simulink model "Lab5_1"  (R2023a)
settings: Solver=FixedStepDiscrete  StartTime=0.0  StopTime=A.len*16 + 52  FixedStep=1  RelTol=1e-3
PostLoadFcn:
  | A = DEScfg_axi('$0102040810204080', 'This is a default input - make it your own!', 'encrypt')
undefined symbols (not defined in the file): AXI4, Lite, xc7z020clg484
libraries: hdlBasic x260, vmcUtilities x1
(part 1 of 2)
settings Model: Creator=gunnarg  LastModifiedBy=robg
settings SolverCC: AlgebraicLoopSolver=TrustRegion
settings DataIOCC: LimitDataPoints=on  SaveFormat=Array  ReturnWorkspaceOutputs=off
settings OptimizationCC: LifeSpan=inf
settings DebuggingCC: SolverPrmCheckMsg=warning  UnconnectedInputMsg=warning  UnconnectedOutputMsg=warning  UnconnectedLineMsg=warning  SFUnexpectedBacktrackingDiag=warning  SFNoUnconditionalDefaultTransitionDiag=warning  ArithmeticOperatorsInVariantConditions=warning
settings HardwareCC: ProdBitPerPointer=32  ProdBitPerSizeT=32  ProdBitPerPtrDiffT=32  ProdLargestAtomicFloat=None  ProdIntDivRoundTo=Undefined  ProdEndianess=Unspecified  ProdWordSize=32  ProdHWDeviceType=32-bit Generic
settings ModelReferenceCC: EnableRefExpFcnMdlSchedulingChecks=on  PropagateSignalLabelsOutOfModel=off
settings SFSimCC: SimUseLocalCustomCode=off  CustomCodeUndefinedFunction=UseInterfaceOnly
settings RTWCC: RTWUseLocalCustomCode=off  DLArmComputeVersion=19.05
settings CodeAppCC: StateflowObjectComments=on
settings GRTTargetCC: TargetLangStandard=C89/C90 (ANSI)
settings ConfigComp: CovMetricSettings=dw  CovSaveCumulativeToWorkspaceVar=on  CovSaveSingleToWorkspaceVar=on  CovExternalEMLEnable=off  CovSFcnEnable=off

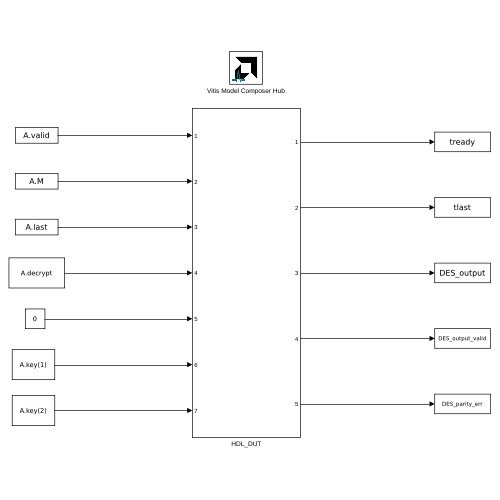
[thumbnail: Simulink's stored preview of the top-level diagram]
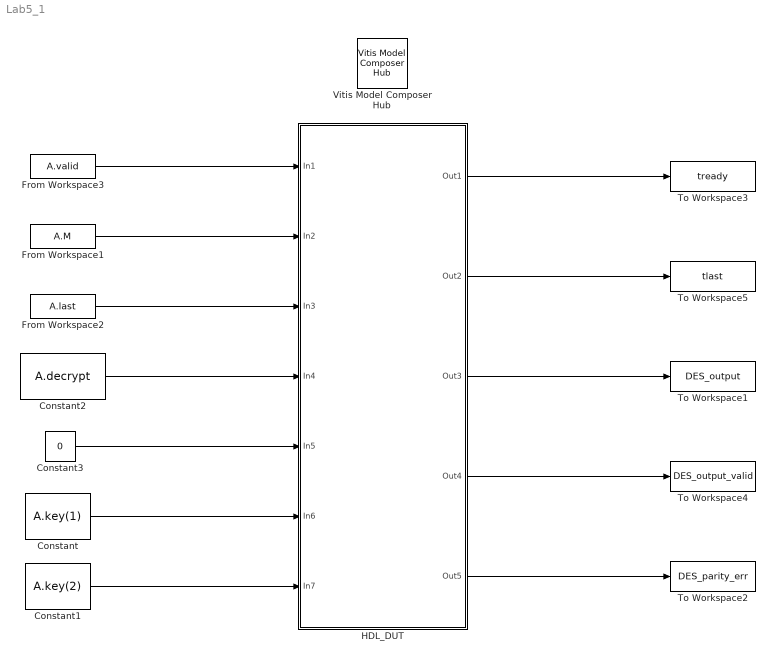
== system Lab5_1 ==
  Constant : Constant  Value=A.key(1)  SampleTime=1
  Constant1 : Constant  Value=A.key(2)  SampleTime=1
  Constant2 : Constant  Value=A.decrypt  VectorParams1D=off
  Constant3 : Constant  Value=0  VectorParams1D=off
  From Workspace1 : FromWorkspace  VariableName=A.M  OutDataTypeStr=uint32  SampleTime=1  Interpolate=off  OutputAfterFinalValue=Setting to zero
  From Workspace2 : FromWorkspace  VariableName=A.last  SampleTime=1  Interpolate=off  OutputAfterFinalValue=Setting to zero
  From Workspace3 : FromWorkspace  VariableName=A.valid  SampleTime=1  Interpolate=off  OutputAfterFinalValue=Setting to zero
  HDL_DUT : Subsystem
  To Workspace1 : ToWorkspace  VariableName=DES_output  SampleTime=-1
  To Workspace2 : ToWorkspace  VariableName=DES_parity_err  SampleTime=-1
  To Workspace3 : ToWorkspace  VariableName=tready  SampleTime=-1
  To Workspace4 : ToWorkspace  VariableName=DES_output_valid  SampleTime=-1
  To Workspace5 : ToWorkspace  VariableName=tlast  SampleTime=-1
  Vitis Model Composer Hub : vmcUtilities/Vitis Model Composer Hub  Tag=genX  CodeGeneration=off  StartColumn=1  NumberOfColumns=1  TargetDirectory=./code  exportDesign=off  analyzeDesign=off  validateDesignOnHw=off  ExportType=System Generator  IpVendor=xilinx.com  IpLibrary=hls  IpVersion=1.0  IpHWLanguage=Verilog  AieCompilerOptions={}  AieSimulatorOptions={}  CreateTestbench=off  TestbenchStackSize=10  RunRtlSim=off  RunCSim=off  RunAieSim=off  AieSimTimeout=50000  RunAieSimProfiling=off  LaunchVitisAnalyzer=off  PlotOutput=off  RunX86Sim=off  X86SimTimeout=10  GenHwImage=off  GenLibadfXo=off  GenHwValidationCode=off  PlatformType=Not Specified  HwSystemType=Baremetal  HwValidationTarget=hw  ProjDevice=xc7z020clg484-1  ProjDevicePart=xc7z020clg484-1  SamplePeriod=-1  ClockFrequency=200  DataPathParallelism=1  xilinxfamily=zynq  part=xc7z020  speed=-1  package=clg484  directory=./IPI_Project  testbench=off  incr_netlist=off  synthesis_tool=Vivado  clock_wrapper=Clock Enables  dbl_ovrd=According to Block Masks  dcm_input_clock_period=10  sysclk_period=10  simulink_period=1  eval_field=0  LogFileName=''  NThreads=4
  wires:
  From Workspace3/1 -> HDL_DUT/1(In1)
  From Workspace1/1 -> HDL_DUT/2(In2)
  From Workspace2/1 -> HDL_DUT/3(In3)
  Constant2/1 -> HDL_DUT/4(In4)
  Constant3/1 -> HDL_DUT/5(In5)
  Constant/1 -> HDL_DUT/6(In6)
  Constant1/1 -> HDL_DUT/7(In7)
  HDL_DUT/1(Out1) -> To Workspace3/1
  HDL_DUT/2(Out2) -> To Workspace5/1
  HDL_DUT/3(Out3) -> To Workspace1/1
  HDL_DUT/4(Out4) -> To Workspace4/1
  HDL_DUT/5(Out5) -> To Workspace2/1

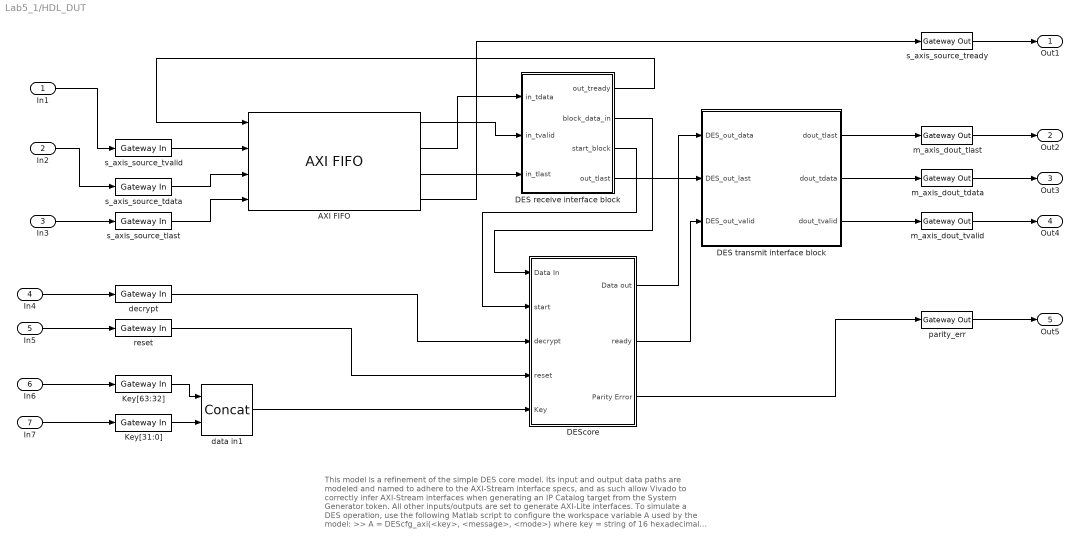
== system Lab5_1/HDL_DUT ==
  note: This model is a refinement of the simple DES core model. Its input and output data paths
      | are modeled and named to adhere to the AXI-Stream interface specs, and as such allow
      | Vivado to correctly infer AXI-Stream interfaces when generating an IP Catalog target from
      | the System Generator token. All other inputs/outputs are set to generate AXI-Lite interfaces.
      |
      | To simulate a DES operation, use the following Matlab script to configure the workspace
      | variable A used by the model:
      | 	>> A = DEScfg_axi(<key>, <message>, <mode>)
      | where
      | 	key = string of 16 hexadecimal digits (prefixes "$" and "0x" are stripped)
      | 	message = arbitrary length string
      | 	mode = either 'encrypt' or 'decrypt'
      |
      | To see the output produced by the simulation you can use the utility function 'DES_print':
      | 	>> DES_print(DES_output, DES_output_valid, tlast)
      |
      | The function will strip all non-valid output (valid signal not asserted)
  In1 : Inport
  In2 : Inport  Port=2
  In3 : Inport  Port=3
  In4 : Inport  Port=4
  In5 : Inport  Port=5
  In6 : Inport  Port=6
  In7 : Inport  Port=7
  AXI FIFO : hdlBasic/AXI FIFO  input_depth_axis=1K  actual_fifo_depth_label=1026  enable_tdata=on  enable_tdest=off  enable_tstrb=off  enable_tready=on  enable_tid=off  enable_tuser=off  enable_tkeep=off  enable_tlast=on  has_aresetn=off  enable_data_counts_axis=off  fifo_implementation_type_axis=Common Clock Block RAM  trim_axipin_name=on  programmable_full_type_axis=Full  full_threshold_assert_value_axis=0  programmable_empty_type_axis=Empty  empty_threshold_assert_value_axis=1022  underflow_flag_axi=0  underflow_sense_axi=Active High  overflow_flag_axi=0  overflow_sense_axi=Active High  simulation_type=fast_sim  XmcBlockStatus=1  maskContainerNames=tabcontainer1  block_type=axi_fifo  block_config=sysgen:AXI_FIFO_config
  DES receive interface block : Subsystem
  DES transmit interface block : Subsystem
  DEScore : Subsystem
  Key[31:0] : hdlBasic/Gateway In  gui_display_data_type=Fixed-point  arith_type=Unsigned  n_bits=32  bin_pt=0  preci_type=Single  exp_width=8  frac_width=24  rows=1  columns=1  quantization=Truncate  overflow=Saturate  period=1  UseAsADC=off  ADCChannel='1'  interface=AXI4-Lite  automatic_assignment=on  address_offset=hex2dec('00')  intf_name=''  intf_description=''  default_value=0  timing_constraint=None  locs_specified=off  LOCs={}  io_standard={}  inherit_from_input=off  hdl_port=on  XmcBlockStatus=1  maskContainerNames=group4  block_type=gatewayin  block_config=sysgen:gateway_in_config  block_width_w=590  block_height_w=620  block_width=640  block_height=850
  Key[63:32] : hdlBasic/Gateway In  gui_display_data_type=Fixed-point  arith_type=Unsigned  n_bits=32  bin_pt=0  preci_type=Single  exp_width=8  frac_width=24  rows=1  columns=1  quantization=Truncate  overflow=Wrap  period=1  UseAsADC=off  ADCChannel='1'  interface=AXI4-Lite  automatic_assignment=on  address_offset=hex2dec('00')  intf_name=''  intf_description=''  default_value=0  timing_constraint=None  locs_specified=off  LOCs={}  io_standard={}  inherit_from_input=off  hdl_port=on  XmcBlockStatus=1  maskContainerNames=group4  block_type=gatewayin  block_config=sysgen:gateway_in_config  block_width_w=590  block_height_w=620  block_width=640  block_height=850
  data in1 : hdlBasic/Concat  num_inputs=2  XmcBlockStatus=1  maskContainerNames=group1  block_type=concat  block_config=sysgen:Concat_config
  decrypt : hdlBasic/Gateway In  gui_display_data_type=Boolean  arith_type=Boolean  n_bits=16  bin_pt=14  preci_type=Single  exp_width=8  frac_width=24  rows=1  columns=1  quantization="Round  (unbiased: +/- Inf)"  overflow=Saturate  period=1  UseAsADC=off  ADCChannel='1'  interface=AXI4-Lite  automatic_assignment=on  address_offset=hex2dec('00')  intf_name=''  intf_description=''  default_value=0  timing_constraint=None  locs_specified=off  LOCs={}  io_standard={}  inherit_from_input=off  hdl_port=on  XmcBlockStatus=1  maskContainerNames=group4  block_type=gatewayin  block_config=sysgen:gateway_in_config  block_width_w=590  block_height_w=620  block_width=640  block_height=850
  m_axis_dout_tdata : hdlBasic/Gateway Out  inherit_from_input=on  hdl_port=on  rows=1  columns=1  UseAsDAC=off  DACChannel='1'  interface=None  automatic_assignment=on  address_offset=hex2dec('00')  intf_name=''  intf_description=''  timing_constraint=None  locs_specified=off  LOCs={}  io_standard={}  XmcBlockStatus=1  maskContainerNames=group4  block_type=gatewayout  block_config=sysgen:gateway_out_config  block_width_w=590  block_height_w=620  block_width=620  block_height=750
  m_axis_dout_tlast : hdlBasic/Gateway Out  inherit_from_input=on  hdl_port=on  rows=1  columns=1  UseAsDAC=off  DACChannel='1'  interface=None  automatic_assignment=on  address_offset=hex2dec('00')  intf_name=''  intf_description=''  timing_constraint=None  locs_specified=off  LOCs={}  io_standard={}  XmcBlockStatus=1  maskContainerNames=group4  block_type=gatewayout  block_config=sysgen:gateway_out_config  block_width_w=590  block_height_w=620  block_width=620  block_height=750
  m_axis_dout_tvalid : hdlBasic/Gateway Out  inherit_from_input=on  hdl_port=on  rows=1  columns=1  UseAsDAC=off  DACChannel='1'  interface=None  automatic_assignment=on  address_offset=hex2dec('00')  intf_name=''  intf_description=''  timing_constraint=None  locs_specified=off  LOCs={}  io_standard={}  XmcBlockStatus=1  maskContainerNames=group4  block_type=gatewayout  block_config=sysgen:gateway_out_config  block_width_w=590  block_height_w=620  block_width=620  block_height=750
  parity_err : hdlBasic/Gateway Out  inherit_from_input=on  hdl_port=on  rows=1  columns=1  UseAsDAC=off  DACChannel='1'  interface=AXI4-Lite  automatic_assignment=on  address_offset=hex2dec('00')  intf_name=''  intf_description=''  timing_constraint=None  locs_specified=off  LOCs={}  io_standard={}  XmcBlockStatus=1  maskContainerNames=group4  block_type=gatewayout  block_config=sysgen:gateway_out_config  block_width_w=590  block_height_w=620  block_width=620  block_height=750
  reset : hdlBasic/Gateway In  gui_display_data_type=Boolean  arith_type=Boolean  n_bits=16  bin_pt=14  preci_type=Single  exp_width=8  frac_width=24  rows=1  columns=1  quantization="Round  (unbiased: +/- Inf)"  overflow=Saturate  period=1  UseAsADC=off  ADCChannel='1'  interface=AXI4-Lite  automatic_assignment=on  address_offset=hex2dec('00')  intf_name=''  intf_description=''  default_value=0  timing_constraint=None  locs_specified=off  LOCs={}  io_standard={}  inherit_from_input=off  hdl_port=on  XmcBlockStatus=1  maskContainerNames=group4  block_type=gatewayin  block_config=sysgen:gateway_in_config  block_width_w=590  block_height_w=620  block_width=640  block_height=850
  s_axis_source_tdata : hdlBasic/Gateway In  gui_display_data_type=Fixed-point  arith_type=Unsigned  n_bits=32  bin_pt=0  preci_type=Single  exp_width=8  frac_width=24  rows=1  columns=1  quantization=Truncate  overflow=Saturate  period=1  UseAsADC=off  ADCChannel='1'  interface=None  automatic_assignment=on  address_offset=hex2dec('00')  intf_name=''  intf_description=''  default_value=0  timing_constraint=None  locs_specified=off  LOCs={}  io_standard={}  inherit_from_input=off  hdl_port=on  XmcBlockStatus=1  maskContainerNames=group4  block_type=gatewayin  block_config=sysgen:gateway_in_config  block_width_w=590  block_height_w=620  block_width=640  block_height=850
  s_axis_source_tlast : hdlBasic/Gateway In  gui_display_data_type=Boolean  arith_type=Boolean  n_bits=32  bin_pt=0  preci_type=Single  exp_width=8  frac_width=24  rows=1  columns=1  quantization=Truncate  overflow=Saturate  period=1  UseAsADC=off  ADCChannel='1'  interface=None  automatic_assignment=on  address_offset=hex2dec('00')  intf_name=''  intf_description=''  default_value=0  timing_constraint=None  locs_specified=off  LOCs={}  io_standard={}  inherit_from_input=off  hdl_port=on  XmcBlockStatus=1  maskContainerNames=group4  block_type=gatewayin  block_config=sysgen:gateway_in_config  block_width_w=590  block_height_w=620  block_width=640  block_height=850
  s_axis_source_tready : hdlBasic/Gateway Out  inherit_from_input=on  hdl_port=on  rows=1  columns=1  UseAsDAC=off  DACChannel='1'  interface=None  automatic_assignment=on  address_offset=hex2dec('00')  intf_name=''  intf_description=''  timing_constraint=None  locs_specified=off  LOCs={}  io_standard={}  XmcBlockStatus=1  maskContainerNames=group4  block_type=gatewayout  block_config=sysgen:gateway_out_config  block_width_w=590  block_height_w=620  block_width=620  block_height=750
  s_axis_source_tvalid : hdlBasic/Gateway In  gui_display_data_type=Boolean  arith_type=Boolean  n_bits=32  bin_pt=0  preci_type=Single  exp_width=8  frac_width=24  rows=1  columns=1  quantization=Truncate  overflow=Saturate  period=1  UseAsADC=off  ADCChannel='1'  interface=None  automatic_assignment=on  address_offset=hex2dec('00')  intf_name=''  intf_description=''  default_value=0  timing_constraint=None  locs_specified=off  LOCs={}  io_standard={}  inherit_from_input=off  hdl_port=on  XmcBlockStatus=1  maskContainerNames=group4  block_type=gatewayin  block_config=sysgen:gateway_in_config  block_width_w=590  block_height_w=620  block_width=640  block_height=850
  Out1 : Outport
  Out2 : Outport  Port=2
  Out3 : Outport  Port=3
  Out4 : Outport  Port=4
  Out5 : Outport  Port=5
  wires:
  AXI FIFO/1 -> DES receive interface block/2(in_tvalid)
  DES transmit interface block/3(dout_tvalid) -> m_axis_dout_tvalid/1
  m_axis_dout_tdata/1 -> Out3/1
  DES transmit interface block/2(dout_tdata) -> m_axis_dout_tdata/1
  DEScore/2(ready) -> DES transmit interface block/3(DES_out_valid)
  data in1/1 -> DEScore/5(Key)
  Key[31:0]/1 -> data in1/2
  DES receive interface block/2(block_data_in) -> DEScore/1(Data In)
  AXI FIFO/4 -> s_axis_source_tready/1
  In3/1 -> s_axis_source_tlast/1
  In1/1 -> s_axis_source_tvalid/1
  parity_err/1 -> Out5/1
  DES receive interface block/4(out_tlast) -> DES transmit interface block/2(DES_out_last)
  Key[63:32]/1 -> data in1/1
  In6/1 -> Key[63:32]/1
  m_axis_dout_tvalid/1 -> Out4/1
  In7/1 -> Key[31:0]/1
  s_axis_source_tdata/1 -> AXI FIFO/3
  DEScore/3(Parity Error) -> parity_err/1
  s_axis_source_tvalid/1 -> AXI FIFO/2
  DES transmit interface block/1(dout_tlast) -> m_axis_dout_tlast/1
  reset/1 -> DEScore/4(reset)
  m_axis_dout_tlast/1 -> Out2/1
  In5/1 -> reset/1
  DEScore/1(Data out) -> DES transmit interface block/1(DES_out_data)
  In4/1 -> decrypt/1
  In2/1 -> s_axis_source_tdata/1
  AXI FIFO/3 -> DES receive interface block/3(in_tlast)
  DES receive interface block/1(out_tready) -> AXI FIFO/1
  AXI FIFO/2 -> DES receive interface block/1(in_tdata)
  s_axis_source_tlast/1 -> AXI FIFO/4
  s_axis_source_tready/1 -> Out1/1
  decrypt/1 -> DEScore/3(decrypt)
  DES receive interface block/3(start_block) -> DEScore/2(start)

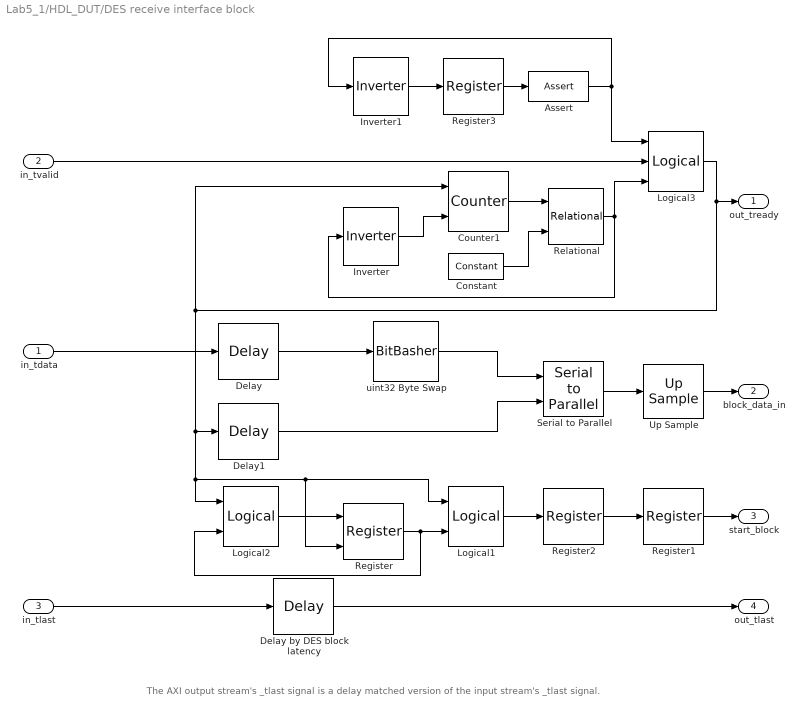
== system Lab5_1/HDL_DUT/DES receive interface block ==
  note: The AXI output stream's _tlast signal is a delay matched version of the input stream's _tlast signal.
  in_tdata : Inport
  in_tvalid : Inport  Port=2
  in_tlast : Inport  Port=3
  Assert : hdlBasic/Assert  assert_type=on  type_source=Explicitly  gui_display_data_type=Boolean  arith_type=Boolean  n_bits=16  bin_pt=14  preci_type=Single  exp_width=8  frac_width=24  assert_rate=on  rate_source=Explicitly  period=1  output_port=on  XmcBlockStatus=1  maskContainerNames=group1  block_type=assert  block_config=sysgen:assert_config  block_width=609  block_height=900
  Constant : hdlBasic/Constant  const=7  gui_display_data_type=Fixed-point  arith_type=Unsigned  n_bits=3  bin_pt=0  preci_type=Single  exp_width=8  frac_width=24  explicit_period=on  period=1  XmcBlockStatus=1  maskContainerNames=tabcontainer1  block_type=constant  block_config=sysgen:Constant_config
  Counter1 : hdlBasic/Counter  cnt_type=Free running  cnt_to=7  operation=Up  start_count=0  cnt_by_val=1  arith_type=Unsigned  n_bits=3  bin_pt=0  load_pin=off  rst=on  en=on  explicit_period=Explicit  period=1  use_behavioral_HDL=off  implementation=Fabric  XmcBlockStatus=1  maskContainerNames=group1  block_type=counter  block_config=sysgen:Counter_config  block_width=531  block_height=1023
  Delay : hdlBasic/Delay  rst=off  en=off  latency=1  reg_retiming=off  XmcBlockStatus=1  maskContainerNames=group1  block_type=delay  block_config=sysgen:Delay_config
  Delay by DES block latency : hdlBasic/Delay  rst=off  en=off  latency=28  reg_retiming=off  XmcBlockStatus=1  maskContainerNames=group1  block_type=delay  block_config=sysgen:Delay_config
  Delay1 : hdlBasic/Delay  rst=off  en=off  latency=1  reg_retiming=off  XmcBlockStatus=1  maskContainerNames=group1  block_type=delay  block_config=sysgen:Delay_config
  Inverter : hdlBasic/Inverter  en=off  latency=0  XmcBlockStatus=1  maskContainerNames=group2  block_type=inv  block_config=sysgen:Inverter_config
  Inverter1 : hdlBasic/Inverter  en=off  latency=0  XmcBlockStatus=1  maskContainerNames=group2  block_type=inv  block_config=sysgen:Inverter_config
  Logical1 : hdlBasic/Logical  logical_function=AND  inputs=2  en=off  latency=0  precision=Full  arith_type=Unsigned  n_bits=16  bin_pt=0  align_bp=on  overflow=[]  quantization=[]  XmcBlockStatus=1  maskContainerNames=tabcontainer1  block_type=logical  block_config=sysgen:Logical_config
  Logical2 : hdlBasic/Logical  logical_function=XOR  inputs=2  en=off  latency=0  precision=Full  arith_type=Unsigned  n_bits=16  bin_pt=0  align_bp=on  overflow=[]  quantization=[]  XmcBlockStatus=1  maskContainerNames=tabcontainer1  block_type=logical  block_config=sysgen:Logical_config
  Logical3 : hdlBasic/Logical  logical_function=AND  inputs=3  en=off  latency=0  precision=User Defined  arith_type=Boolean  n_bits=16  bin_pt=0  align_bp=on  overflow=[]  quantization=[]  XmcBlockStatus=1  maskContainerNames=tabcontainer1  block_type=logical  block_config=sysgen:Logical_config
  Register : hdlBasic/Register  init=0  rst=off  en=on  XmcBlockStatus=1  maskContainerNames=tabcontainer1  block_type=register  block_config=sysgen:Register_config
  Register1 : hdlBasic/Register  init=0  rst=off  en=off  XmcBlockStatus=1  maskContainerNames=tabcontainer1  block_type=register  block_config=sysgen:Register_config
  Register2 : hdlBasic/Register  init=0  rst=off  en=off  XmcBlockStatus=1  maskContainerNames=tabcontainer1  block_type=register  block_config=sysgen:Register_config
  Register3 : hdlBasic/Register  init=1  rst=off  en=off  XmcBlockStatus=1  maskContainerNames=tabcontainer1  block_type=register  block_config=sysgen:Register_config
  Relational : hdlBasic/Relational  mode=a>=b  op_type=Bool  en=off  latency=0  XmcBlockStatus=1  maskContainerNames=tabcontainer1  block_type=relational  block_config=sysgen:Relational_config
  Serial to Parallel : hdlBasic/Serial to Parallel  input_order=Most Significant Word First  arith_type=Unsigned  output_bits=64  bin_pt=0  rst=off  en=on  latency=1  input_bits=[]  XmcBlockStatus=1  maskContainerNames=group3  block_type=s2p  block_config=sysgen:S2P_config
  Up Sample : hdlBasic/Up Sample  sample_ratio=2  copy_samples=on  en=off  latency=0  XmcBlockStatus=1  maskContainerNames=group1  block_type=usamp  block_config=sysgen:Upsample_config
  uint32 Byte Swap : hdlBasic/BitBasher  bitexpr=out={in[7:0],in[15:8],in[23:16],in[31:24]}  display_expr=off  sr_1=out  arith_type1=Unsigned  bin_pt1=0  sr_2=2  arith_type2=Unsigned  bin_pt2=0  sr_3=3  arith_type3=Unsigned  bin_pt3=0  sr_4=4  arith_type4=Unsigned  bin_pt4=0  XmcBlockStatus=1  maskContainerNames=group1  block_type=bitbasher  block_config=sysgen:BitBasher_config
  out_tready : Outport  VectorParamsAs1DForOutWhenUnconnected=off
  block_data_in : Outport  Port=2  VectorParamsAs1DForOutWhenUnconnected=off
  start_block : Outport  Port=3  VectorParamsAs1DForOutWhenUnconnected=off
  out_tlast : Outport  Port=4  VectorParamsAs1DForOutWhenUnconnected=off
  wires:
  in_tdata/1 -> Delay/1
  Register2/1 -> Register1/1
  Serial to Parallel/1 -> Up Sample/1
  Up Sample/1 -> block_data_in/1
  Register/1 -> Logical1/2, Logical2/2
  Logical2/1 -> Register/1
  Logical1/1 -> Register2/1
  Relational/1 -> Logical3/3, Inverter/1
  Logical3/1 -> Counter1/1, Register/2, Logical1/1, Logical2/1, Delay1/1, out_tready/1
  in_tlast/1 -> Delay by DES block latency/1
  Delay by DES block latency/1 -> out_tlast/1
  Counter1/1 -> Relational/1
  Constant/1 -> Relational/2
  Inverter/1 -> Counter1/2
  in_tvalid/1 -> Logical3/2
  Delay/1 -> uint32 Byte Swap/1
  Delay1/1 -> Serial to Parallel/2
  Register1/1 -> start_block/1
  uint32 Byte Swap/1 -> Serial to Parallel/1
  Inverter1/1 -> Register3/1
  Register3/1 -> Assert/1
  Assert/1 -> Inverter1/1, Logical3/1

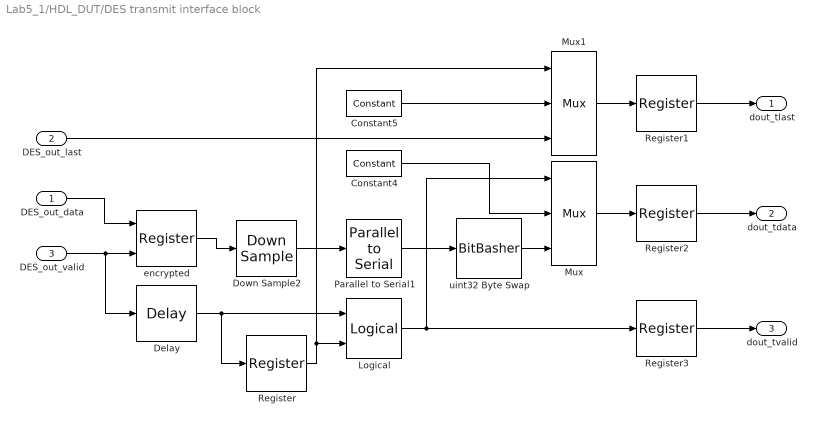
== system Lab5_1/HDL_DUT/DES transmit interface block ==
  DES_out_data : Inport
  DES_out_last : Inport  Port=2
  DES_out_valid : Inport  Port=3
  Constant4 : hdlBasic/Constant  const=0  gui_display_data_type=Fixed-point  arith_type=Unsigned  n_bits=32  bin_pt=0  preci_type=Single  exp_width=8  frac_width=24  explicit_period=on  period=1  XmcBlockStatus=1  maskContainerNames=tabcontainer1  block_type=constant  block_config=sysgen:Constant_config
  Constant5 : hdlBasic/Constant  const=0  gui_display_data_type=Boolean  arith_type=Boolean  n_bits=32  bin_pt=0  preci_type=Single  exp_width=8  frac_width=24  explicit_period=on  period=1  XmcBlockStatus=1  maskContainerNames=tabcontainer1  block_type=constant  block_config=sysgen:Constant_config
  Delay : hdlBasic/Delay  rst=off  en=off  latency=3  reg_retiming=off  XmcBlockStatus=1  maskContainerNames=group1  block_type=delay  block_config=sysgen:Delay_config
  Down Sample2 : hdlBasic/Down Sample  sample_ratio=2  sample_phase="Last Value of Frame  (most efficient)"  en=off  rst=off  latency=1  XmcBlockStatus=1  maskContainerNames=group1  block_type=dsamp  block_config=sysgen:Downsample_config
  Logical : hdlBasic/Logical  logical_function=OR  inputs=2  en=off  latency=0  precision=Full  arith_type=Unsigned  n_bits=16  bin_pt=0  align_bp=on  overflow=[]  quantization=[]  XmcBlockStatus=1  maskContainerNames=tabcontainer1  block_type=logical  block_config=sysgen:Logical_config
  Mux : hdlBasic/Mux  inputs=2  en=off  latency=0  precision=Full  arith_type=Unsigned  n_bits=16  bin_pt=14  quantization=Truncate  overflow=Wrap  XmcBlockStatus=1  maskContainerNames=tabcontainer1  block_type=mux  block_config=sysgen:Mux_config
  Mux1 : hdlBasic/Mux  inputs=2  en=off  latency=0  precision=Full  arith_type=Unsigned  n_bits=16  bin_pt=14  quantization=Truncate  overflow=Wrap  XmcBlockStatus=1  maskContainerNames=tabcontainer1  block_type=mux  block_config=sysgen:Mux_config
  Parallel to Serial1 : hdlBasic/Parallel to Serial  output_order=Most Significant Word First  arith_type=Unsigned  output_bits=32  bin_pt=0  rst=off  en=off  latency=0  XmcBlockStatus=1  maskContainerNames=group1  block_type=p2s  block_config=sysgen:P2S_config
  Register{,1..3} (4 alike) : hdlBasic/Register  init=0  rst=off  en=off  XmcBlockStatus=1  maskContainerNames=tabcontainer1  block_type=register  block_config=sysgen:Register_config
  encrypted : hdlBasic/Register  init=0  rst=off  en=on  XmcBlockStatus=1  maskContainerNames=tabcontainer1  block_type=register  block_config=sysgen:Register_config
  uint32 Byte Swap : hdlBasic/BitBasher  bitexpr=out={in[7:0],in[15:8],in[23:16],in[31:24]}  display_expr=off  sr_1=out  arith_type1=Unsigned  bin_pt1=0  sr_2=2  arith_type2=Unsigned  bin_pt2=0  sr_3=3  arith_type3=Unsigned  bin_pt3=0  sr_4=4  arith_type4=Unsigned  bin_pt4=0  XmcBlockStatus=1  maskContainerNames=group1  block_type=bitbasher  block_config=sysgen:BitBasher_config
  dout_tlast : Outport  VectorParamsAs1DForOutWhenUnconnected=off
  dout_tdata : Outport  Port=2  VectorParamsAs1DForOutWhenUnconnected=off
  dout_tvalid : Outport  Port=3  VectorParamsAs1DForOutWhenUnconnected=off
  wires:
  encrypted/1 -> Down Sample2/1
  Parallel to Serial1/1 -> uint32 Byte Swap/1
  DES_out_data/1 -> encrypted/1
  Constant5/1 -> Mux1/2
  Register3/1 -> dout_tvalid/1
  Register/1 -> Mux1/1, Logical/2
  Constant4/1 -> Mux/2
  Down Sample2/1 -> Parallel to Serial1/1
  DES_out_valid/1 -> Delay/1, encrypted/2
  DES_out_last/1 -> Mux1/3
  Mux/1 -> Register2/1
  Register2/1 -> dout_tdata/1
  Delay/1 -> Logical/1, Register/1
  Mux1/1 -> Register1/1
  Register1/1 -> dout_tlast/1
  Logical/1 -> Mux/1, Register3/1
  uint32 Byte Swap/1 -> Mux/3

== system Lab5_1/HDL_DUT/DEScore ==
  Data In : Inport
  start : Inport  Port=2
  decrypt : Inport  Port=3
  reset : Inport  Port=4
  Key : Inport  Port=5
  DES_fsm : hdlBasic/MCode  mfname=des_ctrl  explicit_period=on  period=1  iptable={'start','';'dec','';'reset',''}  optable={'ctrl','off'}  enable_stdout=off  enable_debug=off  suppress_output=on  defparams={}  hide_port_list={}  block_type=mcode  block_width=444  block_height=788
      settings: infoedit=Pass input values to a MATLAB function for evaluation in Xilinx fixed-point type. The input ports of the block are input arguments of the function. The output ports of the block are output arguments of the function.
  Data : hdlBasic/Register  init=0  rst=off  en=off  XmcBlockStatus=1  maskContainerNames=tabcontainer1  block_type=register  block_config=sysgen:Register_config
  FSM_output : hdlBasic/BitBasher  bitexpr=|  display_expr=off  sr_1=rot2  arith_type1=Unsigned  bin_pt1=0  sr_2=start  arith_type2=Unsigned  bin_pt2=0  sr_3=decrypt  arith_type3=Unsigned  bin_pt3=0  sr_4=4  arith_type4=Unsigned  bin_pt4=0  XmcBlockStatus=1  maskContainerNames=group1  block_type=bitbasher  block_config=sysgen:BitBasher_config
      | <!DOCTYPE HTML PUBLIC "-//W3C//DTD HTML 4.0//EN" "http://www.w3.org/TR/REC-html40/strict.dtd">
      | <html><head><meta name="qrichtext" content="1" /><style type="text/css">
      | p, li { white-space: pre-wrap; }
      | </style></head><body style=" font-family:'MS Shell Dlg 2'; font-size:8.25pt; font-weight:400; font-style:normal;">
      | <p style=" margin-top:12px; margin-bottom:12px; margin-left:0px; margin-right:0px; -qt-block-indent:0; text-indent:0px;"><span style=" font-family:'MS Shell Dlg'; font-size:8pt;">rot2={ctrl[0]}<br />start={ctrl[1]}<br />decrypt={ctrl[2]}<br /></span></p></body></html>
  Key Scheduler : Subsystem
  Start : hdlBasic/Register  init=0  rst=off  en=off  XmcBlockStatus=1  maskContainerNames=tabcontainer1  block_type=register  block_config=sysgen:Register_config
  round_datapath : Subsystem
  Data out : Outport  VectorParamsAs1DForOutWhenUnconnected=off
  ready : Outport  Port=2  VectorParamsAs1DForOutWhenUnconnected=off
  Parity Error : Outport  Port=3  VectorParamsAs1DForOutWhenUnconnected=off
  wires:
  FSM_output/3 -> Key Scheduler/4(decrypt)
  Key/1 -> Key Scheduler/3(KeyData)
  FSM_output/2 -> Start/1, Key Scheduler/2(LoadKey)
  Key Scheduler/2(Parity Error) -> Parity Error/1
  Start/1 -> round_datapath/1(start DES)
  decrypt/1 -> DES_fsm/2
  FSM_output/1 -> Key Scheduler/1(Rot2)
  start/1 -> DES_fsm/1
  round_datapath/1(Cipherout) -> Data out/1
  reset/1 -> round_datapath/4(reset), DES_fsm/3
  DES_fsm/1 -> FSM_output/1
  Data/1 -> round_datapath/2(Plaintext in)
  Key Scheduler/1(Round Key) -> round_datapath/3(Sub Key in)
  Data In/1 -> Data/1
  round_datapath/2(ready) -> ready/1

== system Lab5_1/HDL_DUT/DEScore/Key Scheduler ==
  Rot2 : Inport
  LoadKey : Inport  Port=2
  KeyData : Inport  Port=3
  decrypt : Inport  Port=4
  Concat : hdlBasic/Concat  num_inputs=2  XmcBlockStatus=1  maskContainerNames=group1  block_type=concat  block_config=sysgen:Concat_config
  Key Parity Check : Subsystem
  Mux : hdlBasic/Mux  inputs=2  en=off  latency=0  precision=Full  arith_type=Unsigned  n_bits=16  bin_pt=14  quantization=Truncate  overflow=Wrap  XmcBlockStatus=1  maskContainerNames=tabcontainer1  block_type=mux  block_config=sysgen:Mux_config
  Mux1 : hdlBasic/Mux  inputs=2  en=off  latency=0  precision=Full  arith_type=Unsigned  n_bits=16  bin_pt=14  quantization=Truncate  overflow=Wrap  XmcBlockStatus=1  maskContainerNames=tabcontainer1  block_type=mux  block_config=sysgen:Mux_config
  PC-1 : hdlBasic/BitBasher  bitexpr=|  display_expr=off  sr_1=left  arith_type1=Unsigned  bin_pt1=0  sr_2=right  arith_type2=Unsigned  bin_pt2=0  sr_3=p  arith_type3=Unsigned  bin_pt3=0  sr_4=4  arith_type4=Unsigned  bin_pt4=0  XmcBlockStatus=1  maskContainerNames=group1  block_type=bitbasher  block_config=sysgen:BitBasher_config
      | <!DOCTYPE HTML PUBLIC "-//W3C//DTD HTML 4.0//EN" "http://www.w3.org/TR/REC-html40/strict.dtd">
      | <html><head><meta name="qrichtext" content="1" /><style type="text/css">
      | p, li { white-space: pre-wrap; }
      | </style></head><body style=" font-family:'MS Shell Dlg 2'; font-size:8.25pt; font-weight:400; font-style:normal;">
      | <p style=" margin-top:0px; margin-bottom:0px; margin-left:0px; margin-right:0px; -qt-block-indent:0; text-indent:0px;"><span style=" font-family:'MS Shell Dlg'; font-size:8pt;">left={a[7],a[15],a[23],a[31],a[39],a[47],a[55],a[63],a[6],a[14],a[22],a[30],a[38],a[46],a[54],a[62],a[5],a[13],a[21],a[29],a[37],a[45],a[53],a[61],a[4],a[12],a[20],a[28]}</span></p>
      | <p style=" margin-top:0px; margin-bottom:0px; margin-left:0px; margin-right:0px; -qt-block-indent:0; text-indent:0px;"><span style=" font-family:'MS Shell Dlg'; font-size:8pt;">right={a[1],a[9],a[17],a[25],a[33],a[41],a[49],a[57],a[2],a[10],a[18],a[26],a[34],a[42],a[50],a[58],a[3],a[11],a[19],a[27],a[35],a[43],a[51],a[59],a[36],a[44],a[52],a[60]}</span></p>
      | <p style="-qt-paragraph-type:empty; margin-top:0px; margin-bottom:0px; margin-left:0px; margin-right:0px; -qt-block-indent:0; text-indent:0px; font-size:8pt;"><br /></p></body></html>
  PC-2 : hdlBasic/BitBasher  bitexpr=|  display_expr=off  sr_1=out  arith_type1=Unsigned  bin_pt1=0  sr_2=2  arith_type2=Unsigned  bin_pt2=0  sr_3=3  arith_type3=Unsigned  bin_pt3=0  sr_4=4  arith_type4=Unsigned  bin_pt4=0  XmcBlockStatus=1  maskContainerNames=group1  block_type=bitbasher  block_config=sysgen:BitBasher_config
      | <!DOCTYPE HTML PUBLIC "-//W3C//DTD HTML 4.0//EN" "http://www.w3.org/TR/REC-html40/strict.dtd">
      | <html><head><meta name="qrichtext" content="1" /><style type="text/css">
      | p, li { white-space: pre-wrap; }
      | </style></head><body style=" font-family:'MS Shell Dlg 2'; font-size:8.25pt; font-weight:400; font-style:normal;">
      | <p style=" margin-top:0px; margin-bottom:0px; margin-left:0px; margin-right:0px; -qt-block-indent:0; text-indent:0px;"><span style=" font-family:'MS Shell Dlg'; font-size:8pt;">out={a[42], a[39], a[45], a[32], a[55], a[51], a[53], a[28], a[41], a[50], a[35], a[46], a[33], a[37], a[44], a[52], a[30], a[48], a[40], a[49], a[29], a[36], a[43], a[54], a[15], a[4], a[25], a[19], a[9], a[1], a[26], a[16], a[5], a[11], a[23], a[8], a[12], a[7], a[17], a[0], a[22], a[3], a[10], a[14], a[6], a[20], a[27], a[24]}</span></p>
      | <p style="-qt-paragraph-type:empty; margin-top:0px; margin-bottom:0px; margin-left:0px; margin-right:0px; -qt-block-indent:0; text-indent:0px; font-family:'MS Shell Dlg'; font-size:8pt;"><br /></p></body></html>
  Register : hdlBasic/Register  init=0  rst=off  en=off  XmcBlockStatus=1  maskContainerNames=tabcontainer1  block_type=register  block_config=sysgen:Register_config
  Register1 : hdlBasic/Register  init=0  rst=off  en=off  XmcBlockStatus=1  maskContainerNames=tabcontainer1  block_type=register  block_config=sysgen:Register_config
  RotateRoundKey : Subsystem
  RotateRoundKey1 : Subsystem
  Round Key : Outport  VectorParamsAs1DForOutWhenUnconnected=off
  Parity Error : Outport  Port=2  VectorParamsAs1DForOutWhenUnconnected=off
  wires:
  RotateRoundKey1/1(data_out) -> Register/1
  PC-1/1 -> Mux/3
  Key Parity Check/1(Out1) -> Parity Error/1
  Register/1 -> Concat/2, Mux1/2
  Rot2/1 -> RotateRoundKey1/1(Rotate2), RotateRoundKey/1(Rotate2)
  PC-1/2 -> Mux1/3
  RotateRoundKey/1(data_out) -> Register1/1
  Mux/1 -> RotateRoundKey/2(data_in)
  KeyData/1 -> Key Parity Check/1(In1), PC-1/1
  Register1/1 -> Mux/2, Concat/1
  LoadKey/1 -> Mux1/1, Mux/1, RotateRoundKey1/4(start), RotateRoundKey/4(start)
  PC-2/1 -> Round Key/1
  Mux1/1 -> RotateRoundKey1/2(data_in)
  Concat/1 -> PC-2/1
  decrypt/1 -> RotateRoundKey1/3(decrypt), RotateRoundKey/3(decrypt)

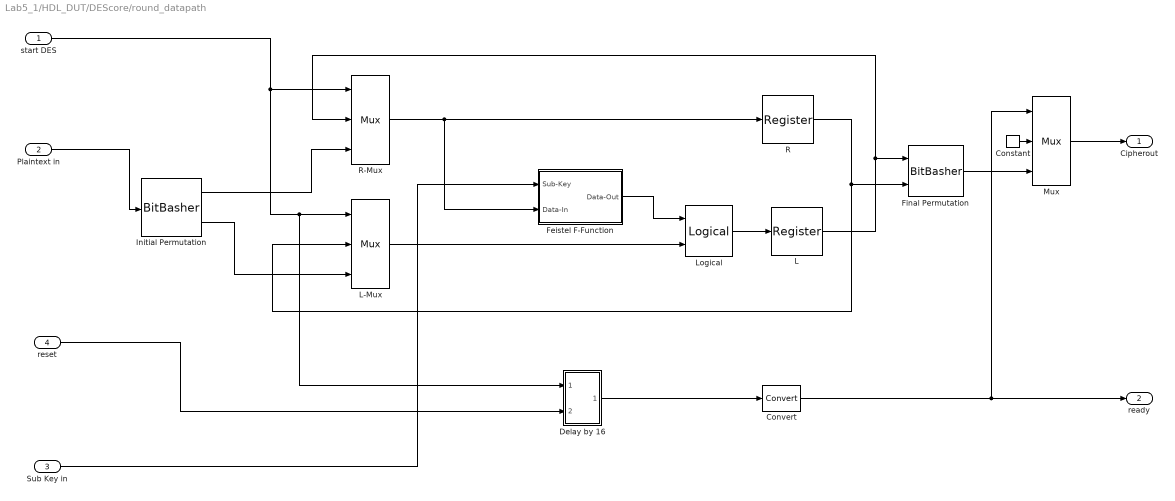
== system Lab5_1/HDL_DUT/DEScore/round_datapath ==
  start DES : Inport
  Plaintext in : Inport  Port=2
  Sub Key in : Inport  Port=3
  reset : Inport  Port=4
  Constant : hdlBasic/Constant  const=0  gui_display_data_type=Fixed-point  arith_type=Unsigned  n_bits=64  bin_pt=0  preci_type=Single  exp_width=8  frac_width=24  explicit_period=on  period=1  XmcBlockStatus=1  maskContainerNames=tabcontainer1  block_type=constant  block_config=sysgen:Constant_config
  Convert : hdlBasic/Convert  gui_display_data_type=Boolean  arith_type=Boolean  n_bits=16  bin_pt=14  float_type=Single  exp_bits=8  fraction_bits=24  quantization=Truncate  overflow=Wrap  en=off  latency=0  pipeline=off  XmcBlockStatus=1  maskContainerNames=group2  block_type=convert  block_config=sysgen:Convert_config  block_width=595  block_height=885
  Delay by 16 : Subsystem
  Feistel F-Function : Subsystem
  Final Permutation : hdlBasic/BitBasher  bitexpr=|  display_expr=off  sr_1=out  arith_type1=Unsigned  bin_pt1=0  sr_2=2  arith_type2=Unsigned  bin_pt2=0  sr_3=3  arith_type3=Unsigned  bin_pt3=0  sr_4=4  arith_type4=Unsigned  bin_pt4=0  XmcBlockStatus=1  maskContainerNames=group1  block_type=bitbasher  block_config=sysgen:BitBasher_config
      | <!DOCTYPE HTML PUBLIC "-//W3C//DTD HTML 4.0//EN" "http://www.w3.org/TR/REC-html40/strict.dtd">
      | <html><head><meta name="qrichtext" content="1" /><style type="text/css">
      | p, li { white-space: pre-wrap; }
      | </style></head><body style=" font-family:'MS Shell Dlg 2'; font-size:8.25pt; font-weight:400; font-style:normal;">
      | <p style=" margin-top:12px; margin-bottom:12px; margin-left:0px; margin-right:0px; -qt-block-indent:0; text-indent:0px;"><span style=" font-family:'MS Shell Dlg'; font-size:8pt;">out={r[24],l[24],r[16],l[16],r[8],l[8],r[0],l[0],r[25],l[25],r[17],l[17],r[9],l[9],r[1],l[1],r[26],l[26],r[18],l[18],r[10],l[10],r[2],l[2],r[27],l[27],r[19],l[19],r[11],l[11],r[3],l[3],r[28],l[28],r[20],l[20],r[12],l[12],r[4],l[4],r[29],l[29],r[21],l[21],r[13],l[13],r[5],l[5],r[30],l[30],r[22],l[22],r[14],l[14],r[6],l[6],r[31],l[31],r[23],l[23],r[15],l[15],r[7],l[7]}</span></p></body></html>
  Initial Permutation : hdlBasic/BitBasher  bitexpr=|  display_expr=off  sr_1=right  arith_type1=Unsigned  bin_pt1=0  sr_2=left  arith_type2=Unsigned  bin_pt2=0  sr_3=3  arith_type3=Unsigned  bin_pt3=0  sr_4=4  arith_type4=Unsigned  bin_pt4=0  XmcBlockStatus=1  maskContainerNames=group1  block_type=bitbasher  block_config=sysgen:BitBasher_config
      | right={in[7],in[15],in[23],in[31],in[39],in[47],in[55],in[63],in[5],in[13],in[21],in[29],in[37],in[45],in[53],in[61],in[3],in[11],in[19],in[27],in[35],in[43],in[51],in[59],in[1],in[9],in[17],in[25],in[33],in[41],in[49],in[57]}
      | left={in[6],in[14],in[22],in[30],in[38],in[46],in[54],in[62],in[4],in[12],in[20],in[28],in[36],in[44],in[52],in[60],in[2],in[10],in[18],in[26],in[34],in[42],in[50],in[58],in[0],in[8],in[16],in[24],in[32],in[40],in[48],in[56]}
  L : hdlBasic/Register  init=0  rst=off  en=off  XmcBlockStatus=1  maskContainerNames=tabcontainer1  block_type=register  block_config=sysgen:Register_config
  L-Mux : hdlBasic/Mux  inputs=2  en=off  latency=0  precision=Full  arith_type=Unsigned  n_bits=16  bin_pt=14  quantization=Truncate  overflow=Wrap  XmcBlockStatus=1  maskContainerNames=tabcontainer1  block_type=mux  block_config=sysgen:Mux_config
  Logical : hdlBasic/Logical  logical_function=XOR  inputs=2  en=off  latency=0  precision=Full  arith_type=Unsigned  n_bits=16  bin_pt=0  align_bp=on  overflow=[]  quantization=[]  XmcBlockStatus=1  maskContainerNames=tabcontainer1  block_type=logical  block_config=sysgen:Logical_config
  Mux : hdlBasic/Mux  inputs=2  en=off  latency=0  precision=Full  arith_type=Unsigned  n_bits=16  bin_pt=14  quantization=Truncate  overflow=Wrap  XmcBlockStatus=1  maskContainerNames=tabcontainer1  block_type=mux  block_config=sysgen:Mux_config
  R : hdlBasic/Register  init=0  rst=off  en=off  XmcBlockStatus=1  maskContainerNames=tabcontainer1  block_type=register  block_config=sysgen:Register_config
  R-Mux : hdlBasic/Mux  inputs=2  en=off  latency=0  precision=Full  arith_type=Unsigned  n_bits=16  bin_pt=14  quantization=Truncate  overflow=Wrap  XmcBlockStatus=1  maskContainerNames=tabcontainer1  block_type=mux  block_config=sysgen:Mux_config
  Cipherout : Outport  VectorParamsAs1DForOutWhenUnconnected=off
  ready : Outport  Port=2  VectorParamsAs1DForOutWhenUnconnected=off
  wires:
  R/1 -> Final Permutation/2, L-Mux/2
  Delay by 16/1(Out1) -> Convert/1
  Feistel F-Function/1(Data-Out) -> Logical/1
  Sub Key in/1 -> Feistel F-Function/1(Sub-Key)
  R-Mux/1 -> Feistel F-Function/2(Data-In), R/1
  start DES/1 -> Delay by 16/1(In1), L-Mux/1, R-Mux/1
  Plaintext in/1 -> Initial Permutation/1
  L/1 -> Final Permutation/1, R-Mux/2
  Logical/1 -> L/1
  Final Permutation/1 -> Mux/3
  L-Mux/1 -> Logical/2
  Initial Permutation/1 -> R-Mux/3
  Initial Permutation/2 -> L-Mux/3
  Convert/1 -> Mux/1, ready/1
  reset/1 -> Delay by 16/2(reset)
  Mux/1 -> Cipherout/1
  Constant/1 -> Mux/2

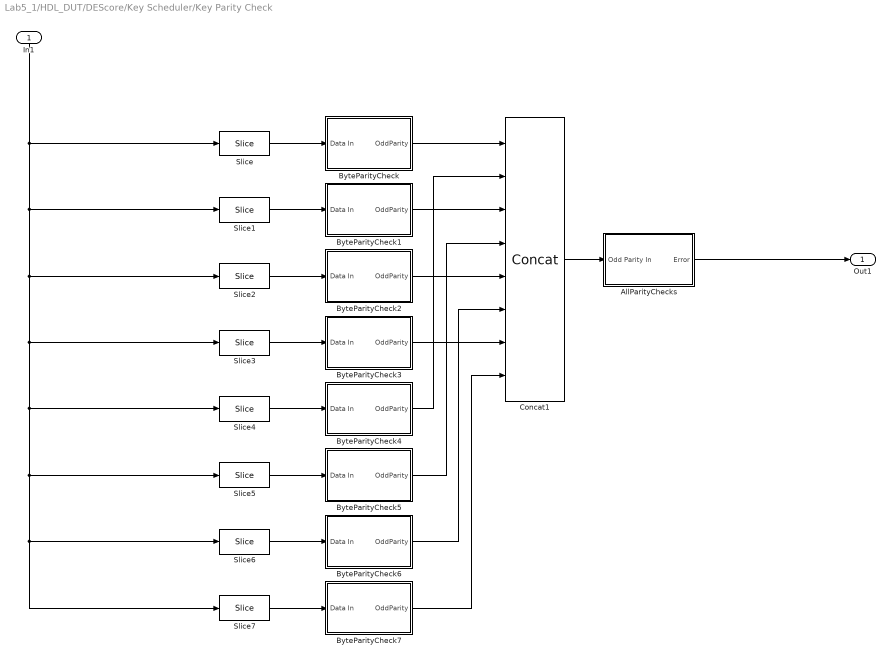
== system Lab5_1/HDL_DUT/DEScore/Key Scheduler/Key Parity Check ==
  In1 : Inport
  AllParityChecks : Subsystem
  ByteParityCheck : Subsystem
  ByteParityCheck1 : Subsystem
  ByteParityCheck2 : Subsystem
  ByteParityCheck3 : Subsystem
  ByteParityCheck4 : Subsystem
  ByteParityCheck5 : Subsystem
  ByteParityCheck6 : Subsystem
  ByteParityCheck7 : Subsystem
  Concat1 : hdlBasic/Concat  num_inputs=8  XmcBlockStatus=1  maskContainerNames=group1  block_type=concat  block_config=sysgen:Concat_config
  Slice : hdlBasic/Slice  nbits=8  boolean_output=off  mode=Lower Bit Location + Width  bit1=0  base1=MSB of Input  bit0=0  base0=LSB of Input  XmcBlockStatus=1  maskContainerNames=group1  block_type=slice  block_config=sysgen:Slice_config
  Slice1 : hdlBasic/Slice  nbits=8  boolean_output=off  mode=Lower Bit Location + Width  bit1=0  base1=MSB of Input  bit0=8  base0=LSB of Input  XmcBlockStatus=1  maskContainerNames=group1  block_type=slice  block_config=sysgen:Slice_config
  Slice2 : hdlBasic/Slice  nbits=8  boolean_output=off  mode=Lower Bit Location + Width  bit1=0  base1=MSB of Input  bit0=16  base0=LSB of Input  XmcBlockStatus=1  maskContainerNames=group1  block_type=slice  block_config=sysgen:Slice_config
  Slice3 : hdlBasic/Slice  nbits=8  boolean_output=off  mode=Lower Bit Location + Width  bit1=0  base1=MSB of Input  bit0=24  base0=LSB of Input  XmcBlockStatus=1  maskContainerNames=group1  block_type=slice  block_config=sysgen:Slice_config
  Slice4 : hdlBasic/Slice  nbits=8  boolean_output=off  mode=Lower Bit Location + Width  bit1=0  base1=MSB of Input  bit0=32  base0=LSB of Input  XmcBlockStatus=1  maskContainerNames=group1  block_type=slice  block_config=sysgen:Slice_config
  Slice5 : hdlBasic/Slice  nbits=8  boolean_output=off  mode=Lower Bit Location + Width  bit1=0  base1=MSB of Input  bit0=40  base0=LSB of Input  XmcBlockStatus=1  maskContainerNames=group1  block_type=slice  block_config=sysgen:Slice_config
  Slice6 : hdlBasic/Slice  nbits=8  boolean_output=off  mode=Lower Bit Location + Width  bit1=0  base1=MSB of Input  bit0=48  base0=LSB of Input  XmcBlockStatus=1  maskContainerNames=group1  block_type=slice  block_config=sysgen:Slice_config
  Slice7 : hdlBasic/Slice  nbits=8  boolean_output=off  mode=Lower Bit Location + Width  bit1=0  base1=MSB of Input  bit0=56  base0=LSB of Input  XmcBlockStatus=1  maskContainerNames=group1  block_type=slice  block_config=sysgen:Slice_config
  Out1 : Outport  VectorParamsAs1DForOutWhenUnconnected=off
  wires:
  ByteParityCheck7/1(OddParity) -> Concat1/8
  ByteParityCheck4/1(OddParity) -> Concat1/2
  ByteParityCheck3/1(OddParity) -> Concat1/7
  ByteParityCheck5/1(OddParity) -> Concat1/4
  Slice6/1 -> ByteParityCheck6/1(Data In)
  Slice5/1 -> ByteParityCheck5/1(Data In)
  Slice4/1 -> ByteParityCheck4/1(Data In)
  Concat1/1 -> AllParityChecks/1(Odd Parity In)
  ByteParityCheck/1(OddParity) -> Concat1/1
  Slice1/1 -> ByteParityCheck1/1(Data In)
  Slice2/1 -> ByteParityCheck2/1(Data In)
  Slice/1 -> ByteParityCheck/1(Data In)
  ByteParityCheck6/1(OddParity) -> Concat1/6
  In1/1 -> Slice/1, Slice1/1, Slice2/1, Slice3/1, Slice4/1, Slice5/1, Slice6/1, Slice7/1
  ByteParityCheck2/1(OddParity) -> Concat1/5
  ByteParityCheck1/1(OddParity) -> Concat1/3
  AllParityChecks/1(Error) -> Out1/1
  Slice7/1 -> ByteParityCheck7/1(Data In)
  Slice3/1 -> ByteParityCheck3/1(Data In)

== system Lab5_1/HDL_DUT/DEScore/Key Scheduler/RotateRoundKey ==
  Rotate2 : Inport
  data_in : Inport  Port=2
  decrypt : Inport  Port=3
  start : Inport  Port=4
  Mux{,1..3} (4 alike) : hdlBasic/Mux  inputs=2  en=off  latency=0  precision=Full  arith_type=Unsigned  n_bits=16  bin_pt=14  quantization=Truncate  overflow=Wrap  XmcBlockStatus=1  maskContainerNames=tabcontainer1  block_type=mux  block_config=sysgen:Mux_config
  ROTL_1 : hdlBasic/BitBasher  bitexpr=|  display_expr=off  sr_1=rotl1  arith_type1=Unsigned  bin_pt1=0  sr_2=2  arith_type2=Unsigned  bin_pt2=0  sr_3=3  arith_type3=Unsigned  bin_pt3=0  sr_4=4  arith_type4=Unsigned  bin_pt4=0  XmcBlockStatus=1  maskContainerNames=group1  block_type=bitbasher  block_config=sysgen:BitBasher_config
      | <!DOCTYPE HTML PUBLIC "-//W3C//DTD HTML 4.0//EN" "http://www.w3.org/TR/REC-html40/strict.dtd">
      | <html><head><meta name="qrichtext" content="1" /><style type="text/css">
      | p, li { white-space: pre-wrap; }
      | </style></head><body style=" font-family:'MS Shell Dlg 2'; font-size:8.25pt; font-weight:400; font-style:normal;">
      | <p style=" margin-top:12px; margin-bottom:12px; margin-left:0px; margin-right:0px; -qt-block-indent:0; text-indent:0px;"><span style=" font-family:'MS Shell Dlg'; font-size:8pt;">rotl1={a[26:0],a[27]}</span></p></body></html>
  ROTL_2 : hdlBasic/BitBasher  bitexpr=|  display_expr=off  sr_1=rotl2  arith_type1=Unsigned  bin_pt1=0  sr_2=2  arith_type2=Unsigned  bin_pt2=0  sr_3=3  arith_type3=Unsigned  bin_pt3=0  sr_4=4  arith_type4=Unsigned  bin_pt4=0  XmcBlockStatus=1  maskContainerNames=group1  block_type=bitbasher  block_config=sysgen:BitBasher_config
      | <!DOCTYPE HTML PUBLIC "-//W3C//DTD HTML 4.0//EN" "http://www.w3.org/TR/REC-html40/strict.dtd">
      | <html><head><meta name="qrichtext" content="1" /><style type="text/css">
      | p, li { white-space: pre-wrap; }
      | </style></head><body style=" font-family:'MS Shell Dlg 2'; font-size:8.25pt; font-weight:400; font-style:normal;">
      | <p style=" margin-top:12px; margin-bottom:12px; margin-left:0px; margin-right:0px; -qt-block-indent:0; text-indent:0px;"><span style=" font-family:'MS Shell Dlg'; font-size:8pt;">rotl2={a[25:0],a[27:26]}</span></p></body></html>
  ROTR_1 : hdlBasic/BitBasher  bitexpr=|  display_expr=off  sr_1=rotr1  arith_type1=Unsigned  bin_pt1=0  sr_2=2  arith_type2=Unsigned  bin_pt2=0  sr_3=3  arith_type3=Unsigned  bin_pt3=0  sr_4=4  arith_type4=Unsigned  bin_pt4=0  XmcBlockStatus=1  maskContainerNames=group1  block_type=bitbasher  block_config=sysgen:BitBasher_config
      | <!DOCTYPE HTML PUBLIC "-//W3C//DTD HTML 4.0//EN" "http://www.w3.org/TR/REC-html40/strict.dtd">
      | <html><head><meta name="qrichtext" content="1" /><style type="text/css">
      | p, li { white-space: pre-wrap; }
      | </style></head><body style=" font-family:'MS Shell Dlg 2'; font-size:8.25pt; font-weight:400; font-style:normal;">
      | <p style=" margin-top:12px; margin-bottom:12px; margin-left:0px; margin-right:0px; -qt-block-indent:0; text-indent:0px;"><span style=" font-family:'MS Shell Dlg'; font-size:8pt;">rotr1={a[0],a[27:1]}</span></p></body></html>
  ROTR_2 : hdlBasic/BitBasher  bitexpr=|  display_expr=off  sr_1=rotr2  arith_type1=Unsigned  bin_pt1=0  sr_2=2  arith_type2=Unsigned  bin_pt2=0  sr_3=3  arith_type3=Unsigned  bin_pt3=0  sr_4=4  arith_type4=Unsigned  bin_pt4=0  XmcBlockStatus=1  maskContainerNames=group1  block_type=bitbasher  block_config=sysgen:BitBasher_config
      | <!DOCTYPE HTML PUBLIC "-//W3C//DTD HTML 4.0//EN" "http://www.w3.org/TR/REC-html40/strict.dtd">
      | <html><head><meta name="qrichtext" content="1" /><style type="text/css">
      | p, li { white-space: pre-wrap; }
      | </style></head><body style=" font-family:'MS Shell Dlg 2'; font-size:8.25pt; font-weight:400; font-style:normal;">
      | <p style=" margin-top:12px; margin-bottom:12px; margin-left:0px; margin-right:0px; -qt-block-indent:0; text-indent:0px;"><span style=" font-family:'MS Shell Dlg'; font-size:8pt;">rotr2={a[1:0],a[27:2]}</span></p></body></html>
  Register : hdlBasic/Register  init=0  rst=off  en=off  XmcBlockStatus=1  maskContainerNames=tabcontainer1  block_type=register  block_config=sysgen:Register_config
  data_out : Outport  VectorParamsAs1DForOutWhenUnconnected=off
  wires:
  Mux1/1 -> data_out/1
  data_in/1 -> Mux3/3, ROTR_1/1, ROTR_2/1, ROTL_2/1, ROTL_1/1
  ROTL_2/1 -> Mux/3
  ROTL_1/1 -> Mux/2
  Rotate2/1 -> Mux/1, Register/1
  ROTR_2/1 -> Mux2/3
  ROTR_1/1 -> Mux2/2
  decrypt/1 -> Mux1/1
  Mux2/1 -> Mux3/2
  Mux/1 -> Mux1/2
  start/1 -> Mux3/1
  Mux3/1 -> Mux1/3
  Register/1 -> Mux2/1
